simulink model "Ue6_Aufgabe1c"  (R2016b)
settings: Solver=VariableStepAuto  StartTime=0.0  StopTime=50000  RelTol=1e-3
undefined symbols (not defined in the file or in its folder): m, n
settings Model: Creator=gome  LastModifiedBy=gome
settings OptimizationCC: LifeSpan=inf
settings DebuggingCC: SFExecutionAtInitializationDiag=none

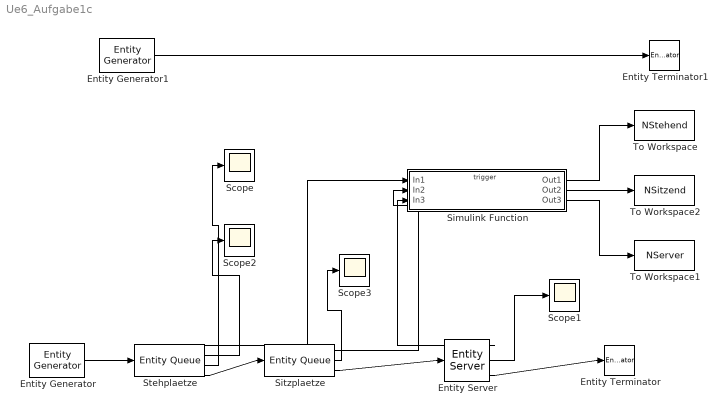
== system Ue6_Aufgabe1c ==
  Entity Generator : EntityGenerator  OutputPortMessageModes=m  TimeSource=MATLAB action  IntergenerationTimeAction=|  EntityType=Structured  EntityTypeName=Entity
      | persistent init
      | if isempty(init)
      |     init = 1;
      |     rng(1);
      | end
      | lambda = 8;
      | dt = exprnd(1/lambda);
  Entity Generator1 : EntityGenerator  OutputPortMessageModes=m  TimeSource=MATLAB action  Period=0.1  IntergenerationTimeAction=|  GenerateAction=getQueueLength  EntityType=Structured  EntityTypeName=Entity
      | persistent init
      | if isempty(init)
      |     init = 1;
      |     rng(23415416);
      | end
      | dt = exprnd(0.1);
  Entity Server : EntityServer  InputPortMessageModes=m  OutputPortMessageModes=n,n,m  Capacity=1  ServiceTimeSource=MATLAB action  ServiceTimeAction=|  NumberEntitiesInBlock=on  Utilization=on
      | persistent init
      | if isempty(init)
      |     init = 1;
      |     rng(4532134);
      | end
      | %mu = 16.9169;
      | mu = 10;
      | dt = exprnd(1/mu);
      settings: OutputPortMap=o1,o5,o9
  Entity Terminator : EntityTerminator  InputPortMessageModes=m
  Entity Terminator1 : EntityTerminator  InputPortMessageModes=m
  Scope{,1..3} (4 alike) : Scope
  Simulink Function : Subsystem  TreatAsAtomicUnit=on
  Sitzplaetze : EntityQueue  InputPortMessageModes=m  OutputPortMessageModes=n,n,m  Capacity=2  NumberEntitiesInBlock=on  AverageWait=on
      settings: OutputPortMap=o1,o2,o5
  Stehplaetze : EntityQueue  InputPortMessageModes=m  OutputPortMessageModes=n,n,n,m  Capacity=inf  NumberEntitiesInBlock=on  AverageWait=on  AverageQueueLength=on
      settings: OutputPortMap=o1,o2,o3,o5
  To Workspace : ToWorkspace  VariableName=NStehend  SampleTime=-1
  To Workspace1 : ToWorkspace  VariableName=NServer  SampleTime=-1
  To Workspace2 : ToWorkspace  VariableName=NSitzend  SampleTime=-1
  wires:
  Entity Generator/1 -> Stehplaetze/1
  Stehplaetze/4 -> Sitzplaetze/1
  Entity Server/3 -> Entity Terminator/1
  Stehplaetze/3 -> Scope/1
  Stehplaetze/1 -> Simulink Function/1(In1)
  Simulink Function/1(Out1) -> To Workspace/1
  Entity Generator1/1 -> Entity Terminator1/1
  Entity Server/2 -> Scope1/1
  Simulink Function/3(Out3) -> To Workspace1/1
  Entity Server/1 -> Simulink Function/3(In3)
  Stehplaetze/2 -> Scope2/1
  Sitzplaetze/3 -> Entity Server/1
  Sitzplaetze/1 -> Simulink Function/2(In2)
  Simulink Function/2(Out2) -> To Workspace2/1
  Sitzplaetze/2 -> Scope3/1

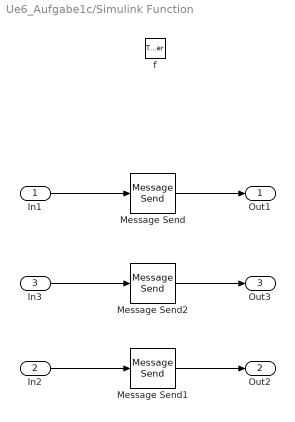
== system Ue6_Aufgabe1c/Simulink Function ==
  In1 : Inport
  In2 : Inport  Port=2
  In3 : Inport  Port=3
  f : TriggerPort  TriggerType=function-call  IsSimulinkFunction=on  FunctionName=getQueueLength  VariantControl=Variant
  Message Send : MessageSend  OutputPortMessageModes=m
      settings: InputPortMap=u1
  Message Send1 : MessageSend  OutputPortMessageModes=m
      settings: InputPortMap=u1
  Message Send2 : MessageSend  OutputPortMessageModes=m
      settings: InputPortMap=u1
  Out1 : Outport
  Out2 : Outport  Port=2
  Out3 : Outport  Port=3
  wires:
  In1/1 -> Message Send/1
  Message Send/1 -> Out1/1
  Message Send1/1 -> Out2/1
  In2/1 -> Message Send1/1
  In3/1 -> Message Send2/1
  Message Send2/1 -> Out3/1
